simulink model "models"  (R2018a)
settings: Solver=VariableStepAuto  StartTime=0.0  StopTime=15  RelTol=1e-3
settings Model: Creator=mmbio  LastModifiedBy=mmbio

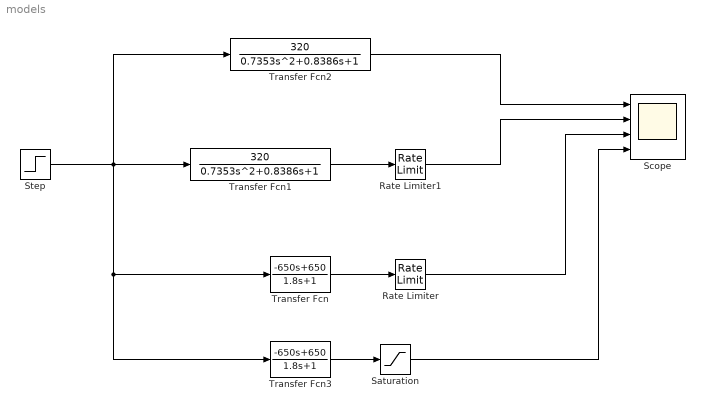
== system models ==
  Rate Limiter : RateLimiter  RisingSlewLimit=190  FallingSlewLimit=0  SampleTimeMode=inherited
  Rate Limiter1 : RateLimiter  RisingSlewLimit=190  FallingSlewLimit=0  SampleTimeMode=inherited
  Saturation : Saturate  UpperLimit=190  LowerLimit=0
  Scope : Scope  NumInputPorts=4
  Step : Step  SampleTime=0
  Transfer Fcn : TransferFcn  Numerator=[-650 650]  Denominator=[1.8 1]
  Transfer Fcn1 : TransferFcn  Numerator=[320]  Denominator=[0.7353 0.8386 1]
  Transfer Fcn2 : TransferFcn  Numerator=[320]  Denominator=[0.7353 0.8386 1]
  Transfer Fcn3 : TransferFcn  Numerator=[-650 650]  Denominator=[1.8 1]
  wires:
  Step/1 -> Transfer Fcn1/1, Transfer Fcn3/1, Transfer Fcn/1, Transfer Fcn2/1
  Transfer Fcn2/1 -> Scope/1
  Transfer Fcn1/1 -> Rate Limiter1/1
  Transfer Fcn/1 -> Rate Limiter/1
  Transfer Fcn3/1 -> Saturation/1
  Saturation/1 -> Scope/4
  Rate Limiter/1 -> Scope/3
  Rate Limiter1/1 -> Scope/2
